simulink model "MATLAB_function"  (R2020a)
settings: Solver=VariableStepAuto  StartTime=0.0  StopTime=10.0  RelTol=1e-3
settings Model: Creator=royde  LastModifiedBy=royde

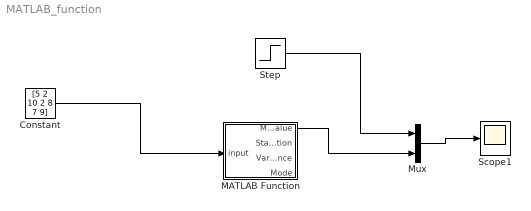
== system MATLAB_function ==
  Constant : Constant  Value=[5 2 10 2 8 7 9]
  MATLAB Function : MATLAB Function  TreatAsAtomicUnit=on
  Mux : Mux  Inputs=2
  Scope1 : Scope
  Step : Step  Before=1  After=10  SampleTime=0
  wires:
  Constant/1 -> MATLAB Function/1(input)
  Step/1 -> Mux/1
  MATLAB Function/1(Mean_value) -> Mux/2
  Mux/1 -> Scope1/1

== matlab function MATLAB_function/MATLAB Function ==
  data: input input; Mean_value output; Standard_deviation output; Variance output; Mode output
function [Mean_value,Standard_deviation,Variance,Mode] = fcn(input)
Mean_value = mean(input);
Standard_deviation = std(input);
Variance = var(input);
Mode = mod(input);
